simulink model "schemat"  (R2021b)
settings: Solver=FixedStepAuto  StartTime=0.0  StopTime=10.0  FixedStep=0.01  RelTol=1e-3
values from neighbouring files (symbols this model uses):
  A = 1    [lab2.m]
  k = 5    [lab2.m]
  p = 0    [lab2.m]
  T = 1    [lab2.m]
  tau = 0    [lab2.m]
  w0 = 5    [lab2.m]
libraries: simulink x1
settings Model: Creator=pc  LastModifiedBy=pc
settings SolverCC: AlgebraicLoopSolver=TrustRegion
settings DebuggingCC: SFMachineParentedDataDiag=warning

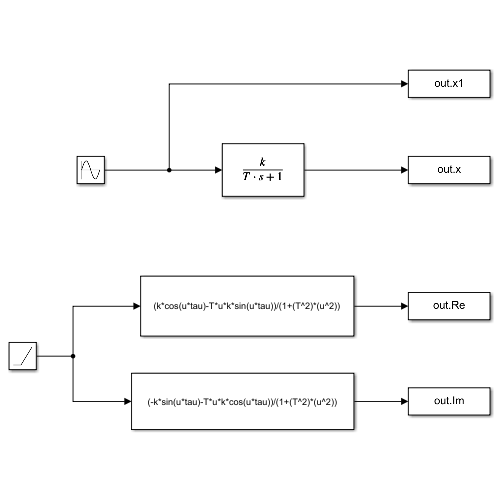
[thumbnail: Simulink's stored preview of the top-level diagram]
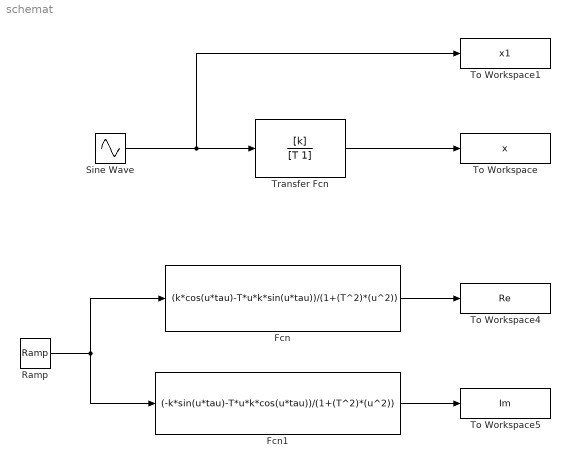
== system schemat ==
  Fcn : Fcn  Expr=(k*cos(u*tau)-T*u*k*sin(u*tau))/(1+(T^2)*(u^2))
  Fcn1 : Fcn  Expr=(-k*sin(u*tau)-T*u*k*cos(u*tau))/(1+(T^2)*(u^2))
  Ramp : simulink/Sources/Ramp  slope=1  start=0  InitialOutput=0
  Sine Wave : Sin  Amplitude=A  Frequency=w0  Phase=p  SampleTime=0
  To Workspace : ToWorkspace  VariableName=x  SampleTime=-1
  To Workspace1 : ToWorkspace  VariableName=x1  SampleTime=-1
  To Workspace4 : ToWorkspace  VariableName=Re  SampleTime=-1
  To Workspace5 : ToWorkspace  VariableName=Im  SampleTime=-1
  Transfer Fcn : TransferFcn  Numerator=[k]  Denominator=[T 1]  ContinuousStateAttributes='position'
  wires:
  Sine Wave/1 -> To Workspace1/1, Transfer Fcn/1
  Transfer Fcn/1 -> To Workspace/1
  Fcn/1 -> To Workspace4/1
  Fcn1/1 -> To Workspace5/1
  Ramp/1 -> Fcn1/1, Fcn/1
